simulink model "rtp_scalar"  (R2019b)
settings: Solver=VariableStepAuto  StartTime=0.0  StopTime=10  RelTol=1e-3
undefined symbols (not defined in the file): S, vsva2197, xcvc1902
libraries: ModelComposer x2
settings Model: Creator=abehbood  LastModifiedBy=viswanad

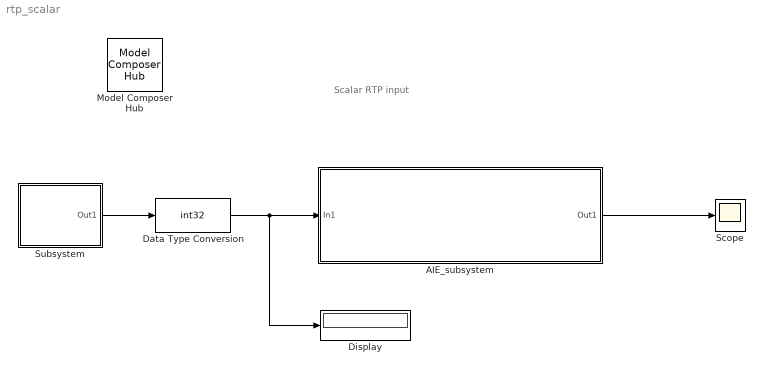
== system rtp_scalar ==
  note: Scalar RTP input
  AIE_subsystem : Subsystem
  Data Type Conversion : DataTypeConversion  OutDataTypeStr=int32
  Display : Display
  Model Composer Hub : ModelComposer/Model Composer Hub  CodeGeneration=off  SubsystemName=AIE_subsystem  TargetDirectory=./code  ExportType=AI Engines  IpVendor=xilinx.com  IpLibrary=hls  IpVersion=1.0  IpHWLanguage=Verilog  AieCompilerOptions={}  CreateTestbench=on  TestbenchStackSize=10  RunAieSim=on  AieSimTimeout=50000  LaunchVitisAnalyzer=off  PlotOutput=off  RunX86Sim=off  X86SimTimeout=10  Platform=xilinx_vck190_base_202110_1  ProjDevice=xcvc1902-vsva2197-2MP-e-S  ProjDevicePart=xcvc1902-vsva2197-2MP-e-S  SamplePeriod=-1  ClockFrequency=200  DataPathParallelism=1
  Scope : Scope
  Subsystem : Subsystem  SystemSampleTime=1  mask(RTP Source){RTP_Value=[10 10 NaN NaN 100 100], SampleTime=1, AfterFinal=Empty}
      mask prompts: RTP_Value "RTP Value:"; SampleTime "Sample Time:"; AfterFinal "Form output after final data:"
      mask help:
      | This block can be used as a source for the RTP input of an AI Engine block. When the RTP input is a scalar, the 'RTP Value' parameter should be a row vector. At each time step, the output is set to one of the elements of the vector starting with the first element. If an element of the vector is NaN, at the corresponding sampling time, the output will be an empty variable-size signal.
      |
      | If the RTP input is a vector, the 'RTP value' parameter should be a matrix. Each column represents an RTP input vector. A NaN column will produce an empty variable-size signal output.
      mask TypeOptions RTP_Value: MATLAB System/RTP_Value
      mask TypeOptions SampleTime: MATLAB System/SampleTime
      mask TypeOptions AfterFinal: MATLAB System/AfterFinal
      mask Display:
      | xmcDrawAIEBlockIcon();
      | disp("RTP Source")
  wires:
  Data Type Conversion/1 -> AIE_subsystem/1(In1), Display/1
  Subsystem/1(Out1) -> Data Type Conversion/1
  AIE_subsystem/1(Out1) -> Scope/1

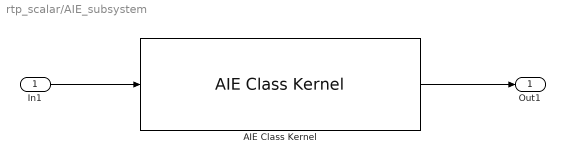
== system rtp_scalar/AIE_subsystem ==
  In1 : Inport
  AIE Class Kernel : ModelComposer/AIE Class Kernel  KernelAllAttrs=|  PortNames={'phase_increment'; 'owin'}  PortSerializedTypes={'{Q1{Bi32}}'; '{P{Toutput_window{1{t{Scint16}}}}}'}  PortWindowSizes={0.000000000000000000e+00; 1.280000000000000000e+02}  PortWindowMargins={0.000000000000000000e+00; 0.000000000000000000e+00}  PortSynchronicities={'sync'; 'auto'}  PortSignalSizes={0.000000000000000000e+00; 0.000000000000000000e+00}  ClassTemplateSpecKind=none  ClassTemplateParamNames={}  ClassTemplateParamKinds={}  ClassTemplateParamTypes={}  ClassTemplateParamValues={}  ClassCtorParamNames={'dds_stored'}  ClassCtorParamSerializedTypes={'{R{Q1{C{Bi16}16}}}'}  ClassCtorParamValues={'[32767 0 32767 0 32767 0 32767 0 32767 0 32767 0 32767 0 32767 0]'}  ClassIndex=1  ClassCtorIndex=1  ClassTabVisible=on  ClassTemplateParamsVisible=off  ClassCtorDeclVisible=on  ClassCtorParamsVisible=on  FunctionTabVisible=on  FunctionDecl=|  PortAttrs={ 'input', 'phase_increment', 'int32 const', '', '', 'sync', ''; 'output', 'owin', 'output_window_cint16 *', '128', '', 'auto', '' }  PortAttrsEnables={'off', 'off', 'off', 'off', 'off', 'on', 'off';'off', 'off', 'off', 'on', 'off', 'on', 'off'}  ClassDeclTypeOptions=C[1 1]@t10@class dds;  ClassDecl=class dds;  ClassTemplateParams={}  ClassTemplateParamsEnables={}  ClassCtorDeclTypeOptions=C[1 1]@t40@dds(int16 const ( & dds_stored ) [ 16 ])  ClassCtorDecl=dds(int16 const ( & dds_stored ) [ 16 ])  ClassCtorParams="{ 'dds_stored', 'int16 const ( &) [ 16 ]', '[32767, 0, 32767, 0, 32767, 0,  32767, 0, 32767, 0, 32767, 0, 32767, 0, 32767, 0]' }"  KernelHeaderFile=src/kernels/dds.h  KernelClassName=dds  KernelFunction=sine  KernelSourceFile=src/kernels/dds.cpp  KernelSearchPaths={}  PreProcOptions={}  CoreRuntimeRatio=0.9  KernelLocSpec=off  ColRowLocation=[0 0]  blockJsonConstraints=[]  deprecateConstraints=0
      KernelAllAttrs=|
      | s[12;12;9;9;19;14;21;23;24;21;12;24;26;26;26;27;28;9;21;23;23;23;24;25;14;19;19;29]@FunctionNameDeclFileNamePortNamesPortTypesPortSerializedTypesPortDirectionsPortWindowSizeEnablesPortWindowMarginEnablesPortSynchronicityEnablesPortSignalSizeEnablesFunctionDeclFunctionTemplateSpecKindFunctionTemplateParamNamesFunctionTemplateParamKindsFunctionTemplateParamTypesFunctionTemplateParamValuesFunctionTemplateParamEnablesClassDeclClassTemplateSpecKindClassTemplateParamNamesClassTemplateParamKindsClassTemplateParamTypesClassTemplateParamValuesClassTemplateParamEnablesClassCtorDeclsClassCtorParamNamesClassCtorParamTypesClassCtorParamSerializedTypes[1 1]@C[28 1]@t4@sinet23@../../src/kernels/dds.hC[2 1]@t15@phase_incrementt4@owinC[2 1]@t11@int32 constt22@output_window_cint16 *C[2 1]@t10@{Q1{Bi32}}t34@{P{Toutput_window{1{t{Scint16}}}}}C[2 1]@t5@inputt6@outputC[2 1]@l0@l1@C[2 1]@l0@l0@C[2 1]@l1@l1@C[2 1]@l0@l0@t73@void dds::
      | sine(int32 const phase_increment, output_window_cint16 * owin)t4@nonee[0 1]@e[0 1]@e[0 1]@e[0 1]@e[0 1]@t10@class dds;t4@nonee[0 1]@e[0 1]@e[0 1]@e[0 1]@e[0 1]@C[1 1]@t40@dds(int16 const ( & dds_stored ) [ 16 ])C[1 1]@C[1 1]@t10@dds_storedC[1 1]@C[1 1]@t23@int16 const ( &) [ 16 ]C[1 1]@C[1 1]@t18@{R{Q1{C{Bi16}16}}}
      FunctionDecl=|
      | void dds::
      | sine(int32 const phase_increment, output_window_cint16 * owin)
  Out1 : Outport
  wires:
  AIE Class Kernel/1 -> Out1/1
  In1/1 -> AIE Class Kernel/1

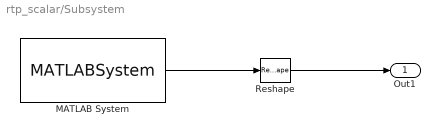
== system rtp_scalar/Subsystem ==
  MATLAB System : MATLABSystem  System=rtp_source  RTP_Value=RTP_Value  SampleTime=SampleTime  AfterFinal=Empty  SimulateUsing=Interpreted execution
      mask Type: rtp_source
      mask Display:
      | disp('rtp_source');
      | port_label('output',1,'rtp');
  Reshape : Reshape
  Out1 : Outport
  wires:
  MATLAB System/1 -> Reshape/1
  Reshape/1 -> Out1/1
